simulink model "gantry_tdg_2025a_karnopp"  (R2025a)
settings: Solver=ode4  StartTime=0.0  StopTime=t(end)  FixedStep=5e-05  RelTol=1e-4  AbsTol=1e-8
undefined symbols (not defined in the file): ca, cb1, cb2, cc1, cc2, ccy, cg1, cg2, cy, d, Jb, Jh, ka, kb1, kb2, L0, Lb, m1, m2, ma, mb, mh, P, ts, Y
libraries: cstblocks x1
settings Model: Creator=cocuser  LastModifiedBy=20203253
settings DataIOCC: ReturnWorkspaceOutputs=off

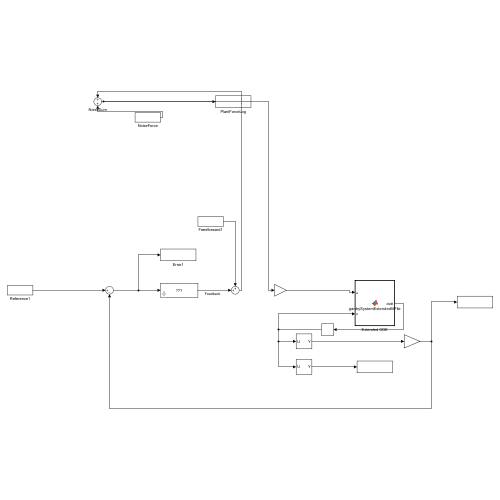
[thumbnail: Simulink's stored preview of the top-level diagram]
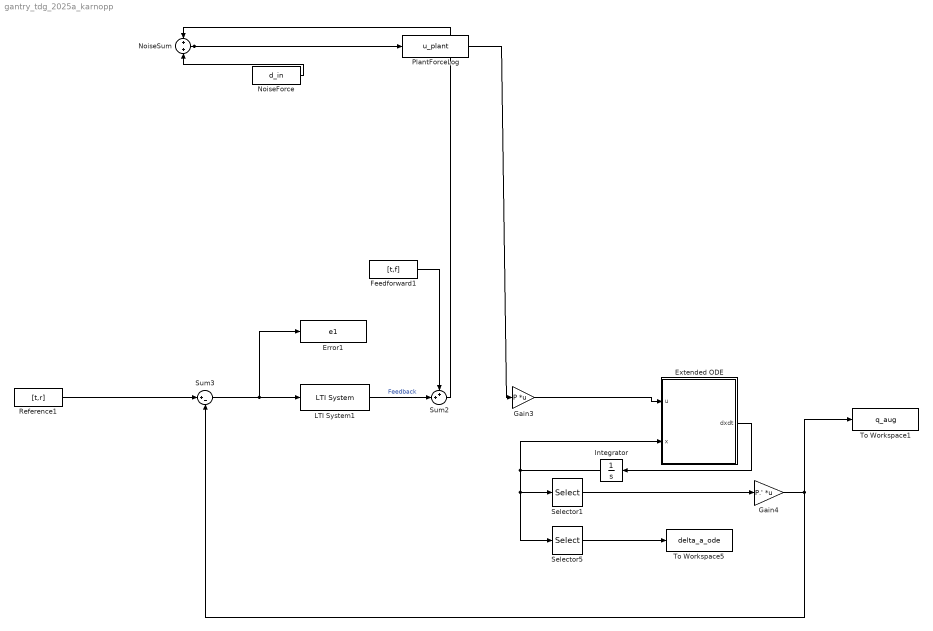
== system gantry_tdg_2025a_karnopp ==
  Error1 : ToWorkspace  VariableName=e1  SampleTime=ts
  Extended ODE : MATLAB Function  TreatAsAtomicUnit=on
  Feedforward1 : FromWorkspace  VariableName=[t,f]  SampleTime=ts
  Gain3 : Gain  Gain=P  Multiplication=Matrix(K*u)
  Gain4 : Gain  Gain=P.'  Multiplication=Matrix(K*u)
  Integrator : Integrator  InitialCondition=[0; 0; Y; 0; 0; 0; 0; 0]
  LTI System1 : cstblocks/LTI System  sys=Cfb  IC=[]  PadeOrder=0
  NoiseForce : FromWorkspace  VariableName=d_in  SampleTime=ts  Interpolate=off  OutputAfterFinalValue=Holding final value
  NoiseSum : Sum
  PlantForceLog : ToWorkspace  VariableName=u_plant  SampleTime=ts
  Reference1 : FromWorkspace  VariableName=[t,r]  SampleTime=ts
  Selector1 : Selector  InputPortWidth=8  IndexOptions=Index vector (dialog)  Indices=[1 2 3]  OutputSizes=1
  Selector5 : Selector  InputPortWidth=8  IndexOptions=Index vector (dialog)  Indices=[4]  OutputSizes=1
  Sum2 : Sum  Inputs=++|
  Sum3 : Sum  Inputs=|+-
  To Workspace1 : ToWorkspace  VariableName=q_aug  SampleTime=ts
  To Workspace5 : ToWorkspace  VariableName=delta_a_ode  SampleTime=ts
  wires:
  LTI System1/1 -> Sum2/2  "Feedback"
  Feedforward1/1 -> Sum2/1
  Sum3/1 -> Error1/1, LTI System1/1
  Selector1/1 -> Gain4/1
  Gain4/1 -> To Workspace1/1, Sum3/2
  Reference1/1 -> Sum3/1
  Gain3/1 -> Extended ODE/1(u)
  Extended ODE/1(dxdt) -> Integrator/1
  Selector5/1 -> To Workspace5/1
  Integrator/1 -> Selector1/1, Selector5/1, Extended ODE/2(x)
  Sum2/1 -> NoiseSum/1
  NoiseForce/1 -> NoiseSum/2
  NoiseSum/1 -> Gain3/1, PlantForceLog/1

== matlab function gantry_tdg_2025a_karnopp/Extended ODE ==
  data: dxdt output; u input; x input; Lb parameter; kb1 parameter; kb2 parameter; m1 parameter; cy parameter; ma parameter; cg2 parameter; cb1 parameter; cg1 parameter; d parameter; Jh parameter; Jb parameter; mh parameter; m2 parameter; ca parameter; mb parameter; cb2 parameter; ka parameter; L0 parameter; cc1 parameter; cc2 parameter; ccy parameter; ts parameter
function dxdt = gantrySystemExtendedMFile(u, x, Lb, kb1, kb2, m1, cy, ma, cg2, cb1, cg1, d, Jh, Jb, mh, m2, ca, mb, cb2, ka, L0, cc1, cc2, ccy, ts)
dxdt = zeros(8,1);
dxdt = gantrySystemExtendedCoulomb(u, x, m1, m2, mb, mh, Lb, Jb, Jh, d, cg1, cg2, cb1, cb2, cy, kb1, kb2, ma, ka, ca, L0, cc1, cc2, ccy, ts);
end
